simulink model "Problem3"  (R2020b)
settings: Solver=VariableStepAuto  StartTime=0.0  StopTime=10.0  RelTol=1e-3
settings Model: Creator=omkar  LastModifiedBy=omkar

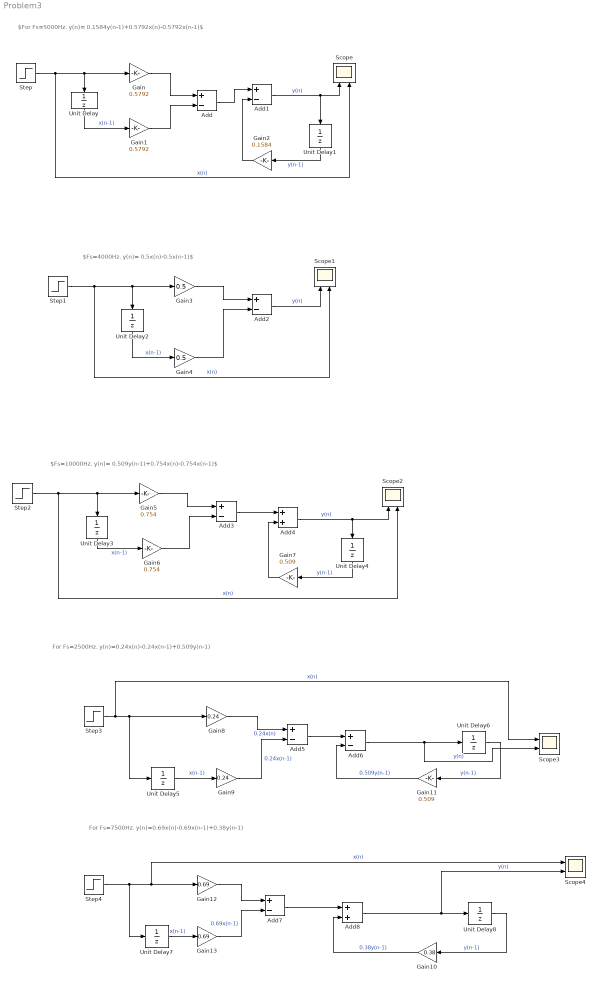
== system Problem3 ==
  note: $For Fs=5000Hz. y(n)= 0.1584y(n-1)+0.5792x(n)-0.5792x(n-1)$
  note: $Fs=4000Hz. y(n)= 0.5x(n)-0.5x(n-1)$
  note: $Fs=10000Hz. y(n)= 0.509y(n-1)+0.754x(n)-0.754x(n-1)$
  note: For Fs=2500Hz. y(n)=0.24x(n)-0.24x(n-1)+0.509y(n-1)
  note: For Fs=7500Hz. y(n)=0.69x(n)-0.69x(n-1)+0.38y(n-1)
  Add{,1..3,5..7} (7 alike) : Sum  Inputs=+-
  Add4 : Sum
  Add8 : Sum
  Gain : Gain  Gain=0.5792
  Gain1 : Gain  Gain=0.5792
  Gain10 : Gain  Gain=0.38
  Gain11 : Gain  Gain=0.509
  Gain12 : Gain  Gain=0.69
  Gain13 : Gain  Gain=0.69
  Gain2 : Gain  Gain=0.1584
  Gain3 : Gain  Gain=0.5
  Gain4 : Gain  Gain=0.5
  Gain5 : Gain  Gain=0.754
  Gain6 : Gain  Gain=0.754
  Gain7 : Gain  Gain=0.509
  Gain8 : Gain  Gain=0.24
  Gain9 : Gain  Gain=0.24
  Scope{,1..4} (5 alike) : Scope  NumInputPorts=2
  Step{,1..4} (5 alike) : Step  SampleTime=0
  Unit Delay{,1..8} (9 alike) : UnitDelay  SampleTime=-1  HasFrameUpgradeWarning=on
  wires:
  Step/1 -> Gain/1, Unit Delay/1, Scope/2  "x(n)"
  Unit Delay/1 -> Gain1/1  "x(n-1)"
  Gain/1 -> Add/1
  Gain1/1 -> Add/2
  Add/1 -> Add1/1
  Unit Delay1/1 -> Gain2/1  "y(n-1)"
  Gain2/1 -> Add1/2
  Add1/1 -> Unit Delay1/1, Scope/1  "y(n)"
  Step1/1 -> Gain3/1, Unit Delay2/1, Scope1/2  "x(n)"
  Unit Delay2/1 -> Gain4/1  "x(n-1)"
  Gain3/1 -> Add2/1
  Gain4/1 -> Add2/2
  Add2/1 -> Scope1/1  "y(n)"
  Step2/1 -> Gain5/1, Unit Delay3/1, Scope2/2  "x(n)"
  Unit Delay3/1 -> Gain6/1  "x(n-1)"
  Gain5/1 -> Add3/1
  Gain6/1 -> Add3/2
  Add3/1 -> Add4/1
  Gain7/1 -> Add4/2
  Add4/1 -> Scope2/1, Unit Delay4/1  "y(n)"
  Unit Delay4/1 -> Gain7/1  "y(n-1)"
  Gain10/1 -> Add8/2  "0.38y(n-1)"
  Unit Delay8/1 -> Gain10/1  "y(n-1)"
  Add8/1 -> Unit Delay8/1, Scope4/2  "y(n)"
  Add7/1 -> Add8/1
  Gain13/1 -> Add7/2  "0.69x(n-1)"
  Gain12/1 -> Add7/1
  Unit Delay7/1 -> Gain13/1  "x(n-1)"
  Step4/1 -> Gain12/1, Scope4/1, Unit Delay7/1  "x(n)"
  Gain11/1 -> Add6/2  "0.509y(n-1)"
  Unit Delay6/1 -> Gain11/1  "y(n-1)"
  Add6/1 -> Unit Delay6/1, Scope3/2  "y(n)"
  Add5/1 -> Add6/1
  Gain8/1 -> Add5/1  "0.24x(n)"
  Gain9/1 -> Add5/2  "0.24x(n-1)"
  Unit Delay5/1 -> Gain9/1  "x(n-1)"
  Step3/1 -> Gain8/1, Unit Delay5/1, Scope3/1  "x(n)"
